simulink model "identifica_srv02l_problem"  (Simulink 7.2)
settings: Solver=ode1  StartTime=0.0  StopTime=3  FixedStep=0.001  RelTol=1e-3  AbsTol=1e-6
values from neighbouring files (symbols this model uses):
  a = param_otim(2)    [calc_all.m]    (also in calc_all_old_v.m; controlador_cal.m = 14.1465; exp1_3.mat = 1; exp1_3_1.mat = 10)
  b = param_otim(1)    [calc_all.m]    (also in calc_all_old_v.m; controlador_cal.m = 4.028; exp1_3.mat = 1; exp1_3_1.mat = 0.825375)
  K_AMP = 1    [exp1_3.mat]    (also in exp1_3_1.mat; exp1_T.mat; exp1_T2.mat; exp1_T3.mat)
  K_ENC = 0.00153398078789    [exp1_3.mat]    (also in exp1_3_1.mat; exp1_T.mat; exp1_T2.mat; exp1_T3.mat)
  K_POT = -0.614355896702    [exp1_3.mat]    (also in exp1_3_1.mat; exp1_T.mat; exp1_T2.mat; exp1_T3.mat)
  K_TACH = -0.99733100114    [exp1_3.mat]    (also in exp1_3_1.mat; exp1_T.mat; exp1_T2.mat; exp1_T3.mat)
  L = 0    [exp1_3.mat]    (also in exp1_3_1.mat = 0.026; exp1_T.mat; exp1_T2.mat; exp1_T3.mat)
  VMAX_AMP = 24    [exp1_3.mat]    (also in exp1_3_1.mat; exp1_T.mat; exp1_T2.mat; exp1_T3.mat)
  VMAX_DAC = 10    [exp1_3.mat]    (also in exp1_3_1.mat; exp1_T.mat; exp1_T2.mat; exp1_T3.mat)
  wcf_e = 157.079632679    [exp1_3.mat]    (also in exp1_3_1.mat; exp1_T.mat; exp1_T2.mat; exp1_T3.mat)
  zetaf_e = 0.9    [exp1_3.mat]    (also in exp1_3_1.mat; exp1_T.mat; exp1_T2.mat; exp1_T3.mat)
undefined symbols (not defined in the file or in its folder): HIL, qc_get_step_size
libraries: quarc_library x4, simulink x1
settings Model: Creator=MLevis  LastModifiedBy=aluno  SimulationMode=external  ExtModeTrigDuration=1000000  BufferReuse=off
settings SolverCC: PositivePriorityOrder=on
settings DataIOCC: LimitDataPoints=off
settings OptimizationCC: BlockReduction=off  BooleanDataType=off  InlineInvariantSignals=on  OptimizeBlockIOStorage=off  BufferReuse=off  ExpressionFolding=off  LocalBlockOutputs=off  InitFltsAndDblsToZero=on
settings DebuggingCC: SaveWithParameterizedLinksMsg=none  SignalResolutionControl=TryResolveAllWithWarning  SolverPrmCheckMsg=none  MultiTaskDSMMsg=warning  MultiTaskCondExecSysMsg=none  StrictBusMsg=None
settings HardwareCC: TargetHWDeviceType=32-bit Generic
settings RTWCC: SystemTargetFile=quarc_windows.tlc  TemplateMakefile=quarc_default_tmf  Description=Quarc Win32 Target  ProcessScript=quarc_windows_make_rtw_hook  IncludeERTFirstTime=on
settings STFCustomTargetCC: TargetFcnLib=ansi_tfl_tmw.mat  TargetPreCompLibLocation=C:\DOCUME~1\ALLUSE~1\DADOSD~1\QUARC\lib\2008b\windows\release  SystemTargetFile=quarc_windows.tlc
settings GRTTargetCC: TargetFcnLib=ansi_tfl_tmw.mat  TargetPreCompLibLocation=C:\DOCUME~1\ALLUSE~1\DADOSD~1\QUARC\lib\2008b\windows\release  CompOptLevelCompliant=off  MatFileLogging=off  ExtMode=on  ExtModeMexFile=quarc_comm

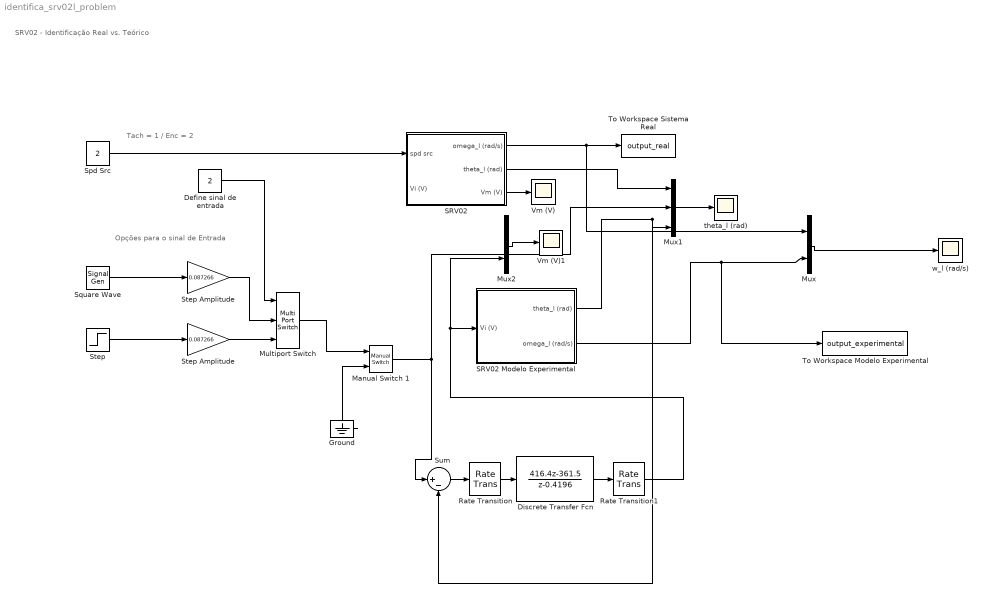
== system identifica_srv02l_problem ==
  note: SRV02 - Identificação
      | Real vs. Teórico
  note: Tach = 1 / Enc = 2
  note: Opções para o sinal de Entrada
  Define sinal de entrada : Constant  Value=2  OutDataType=fixdt(1, 16)  OutScaling=2^0
  Discrete Transfer Fcn : DiscreteTransferFcn  Numerator=[416.4 -361.5]  Denominator=[1 -0.4196]  SampleTime=0.01
  Ground : Ground
  Manual Switch 1 : simulink/Signal Routing/Manual Switch  SystemSampleTime=-1  sw=1  action=0  varsize=off
  Multiport Switch : MultiPortSwitch  Inputs=2  OutDataType=fixdt(1, 16)  OutScaling=2^0
  Mux : Mux  Inputs=2
  Mux1 : Mux  Inputs=3
  Mux2 : Mux  Inputs=2
  Rate Transition : RateTransition  OutPortSampleTime=0.01
  Rate Transition1 : RateTransition  OutPortSampleTime=0.001
  SRV02 : Subsystem
  SRV02 Modelo Experimental : Subsystem
  Spd Src : Constant  Value=2  OutDataType=sfix(16)  OutScaling=2^0
  Square Wave : SignalGenerator  WaveForm=square  Frequency=5
  Step : Step  Time=0.5  SampleTime=0
  Step Amplitude : Gain  Gain=0.087266  ParameterDataType=sfix(16)  ParameterScaling=2^0  OutDataType=sfix(16)  OutScaling=2^0  SaturateOnIntegerOverflow=on  OutDataTypeStr=Inherit: Same as input  ParamDataTypeStr=Inherit: Same as input
  "Step Amplitude " : Gain  Gain=0.087266  ParameterDataType=sfix(16)  ParameterScaling=2^0  OutDataType=sfix(16)  OutScaling=2^0  SaturateOnIntegerOverflow=on  OutDataTypeStr=Inherit: Same as input  ParamDataTypeStr=Inherit: Same as input
  Sum : Sum  Inputs=|+-  OutDataType=sfix(16)  OutScaling=2^0
  To Workspace Modelo Experimental : ToWorkspace  VariableName=output_experimental  SampleTime=-1  SaveFormat=Structure With Time
  To Workspace Sistema Real : ToWorkspace  VariableName=output_real  SampleTime=-1  SaveFormat=Structure With Time
  Vm (V) : Scope
      settings: TimeRange=5  SaveName=Vm  DataFormat=Array
  Vm (V)1 : Scope
      settings: TimeRange=5  SaveName=Vm1  DataFormat=Array
  theta_l (rad) : Scope
      settings: TimeRange=5  YMin=-2.75  YMax=2.75  SaveName=theta  DataFormat=Array
  w_l (rad/s) : Scope
      settings: TimeRange=5  YMin=-2.75  YMax=2.75  SaveName=wl  DataFormat=Array
  wires:
  Mux/1 -> w_l (rad/s)/1
  SRV02/1(omega_l (rad/s)) -> Mux/1, To Workspace Sistema Real/1
  Spd Src/1 -> SRV02/1(spd src)
  Define sinal de entrada/1 -> Multiport Switch/1
  Step/1 -> "Step Amplitude "/1
  Square Wave/1 -> Step Amplitude/1
  "Step Amplitude "/1 -> Multiport Switch/3
  Ground/1 -> Manual Switch 1/2
  SRV02 Modelo Experimental/2(omega_l (rad/s)) -> Mux/2, To Workspace Modelo Experimental/1
  Mux1/1 -> theta_l (rad)/1
  SRV02/2(theta_l (rad)) -> Mux1/1
  SRV02 Modelo Experimental/1(theta_l (rad)) -> Sum/2, Mux1/3
  Multiport Switch/1 -> Manual Switch 1/1
  SRV02/3(Vm (V)) -> Vm (V)/1
  Manual Switch 1/1 -> Sum/1, Mux1/2
  Step Amplitude/1 -> Multiport Switch/2
  Mux2/1 -> Vm (V)1/1
  Sum/1 -> Rate Transition/1
  Rate Transition/1 -> Discrete Transfer Fcn/1
  Discrete Transfer Fcn/1 -> Rate Transition1/1
  Rate Transition1/1 -> SRV02 Modelo Experimental/1(Vi (V)), Mux2/2

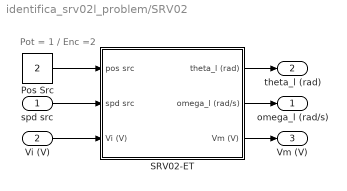
== system identifica_srv02l_problem/SRV02 ==
  note: Pot = 1 / Enc =2
  spd src : Inport  OutDataType=sfix(16)  OutScaling=2^0
  Vi (V) : Inport  Port=2  OutDataType=sfix(16)  OutScaling=2^0
  Pos Src : Constant  Value=2  OutDataType=sfix(16)  OutScaling=2^0
  SRV02-ET : Subsystem
  omega_l (rad/s) : Outport  OutDataType=sfix(16)  OutScaling=2^0
  theta_l (rad) : Outport  Port=2  OutDataType=sfix(16)  OutScaling=2^0
  Vm (V) : Outport  Port=3  OutDataType=sfix(16)  OutScaling=2^0
  wires:
  SRV02-ET/3(Vm (V)) -> Vm (V)/1
  Vi (V)/1 -> SRV02-ET/3(Vi (V))
  SRV02-ET/2(omega_l (rad/s)) -> omega_l (rad/s)/1
  spd src/1 -> SRV02-ET/2(spd src)
  Pos Src/1 -> SRV02-ET/1(pos src)
  SRV02-ET/1(theta_l (rad)) -> theta_l (rad)/1

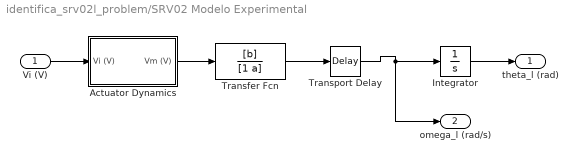
== system identifica_srv02l_problem/SRV02 Modelo Experimental ==
  Vi (V) : Inport  OutDataType=sfix(16)  OutScaling=2^0
  Actuator Dynamics : Subsystem
  Integrator : Integrator
  Transfer Fcn : TransferFcn  Numerator=[b]  Denominator=[1 a]
  Transport Delay : TransportDelay  DelayTime=L
  theta_l (rad) : Outport  OutDataType=sfix(16)  OutScaling=2^0
  omega_l (rad/s) : Outport  Port=2  OutDataType=sfix(16)  OutScaling=2^0
  wires:
  Vi (V)/1 -> Actuator Dynamics/1(Vi (V))
  Actuator Dynamics/1(Vm (V)) -> Transfer Fcn/1
  Integrator/1 -> theta_l (rad)/1
  Transfer Fcn/1 -> Transport Delay/1
  Transport Delay/1 -> Integrator/1, omega_l (rad/s)/1

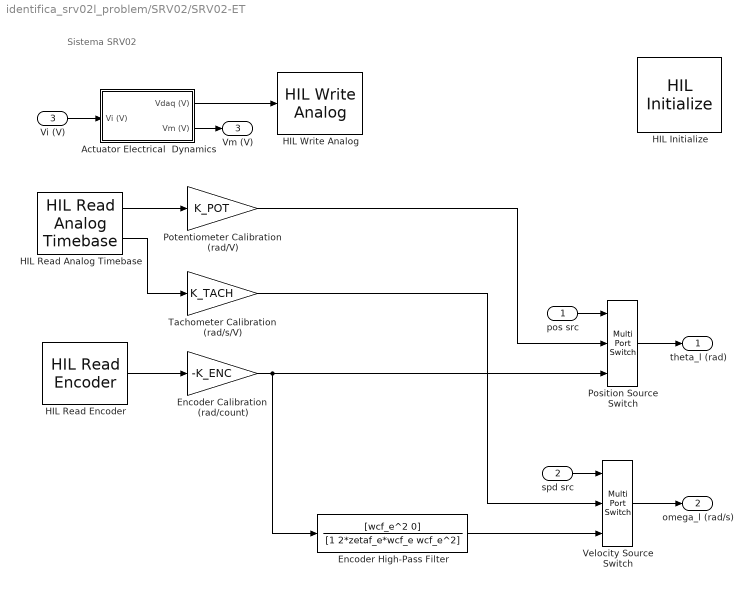
== system identifica_srv02l_problem/SRV02/SRV02-ET ==
  note: Sistema SRV02
  pos src : Inport  OutDataType=sfix(16)  OutScaling=2^0
  spd src : Inport  Port=2  OutDataType=sfix(16)  OutScaling=2^0
  Vi (V) : Inport  Port=3  OutDataType=sfix(16)  OutScaling=2^0
  Actuator Electrical  Dynamics : Subsystem
  Encoder Calibration  (rad/count) : Gain  Gain=-K_ENC  ParameterDataType=sfix(16)  ParameterScaling=2^0  OutDataType=sfix(16)  OutScaling=2^0  SaturateOnIntegerOverflow=on  OutDataTypeStr=Inherit: Same as input  ParamDataTypeStr=Inherit: Same as input
  Encoder High-Pass Filter : TransferFcn  Numerator=[wcf_e^2 0]  Denominator=[1 2*zetaf_e*wcf_e wcf_e^2]
  HIL Initialize : quarc_library/Data Acquisition/Generic/Configuration/HIL Initialize  object_name=HIL-1  board_type=q8_usb  board_number=0  board_options=update_rate=normal  exclusive=off  active=off  hardware_clocks=[0:2]  clock_modes=[]  set_clock_params_at_start=off  set_clock_params_at_switch_in=off  analog_input_channels=[0:7]  analog_input_maximums=10  analog_input_minimums=-10  set_analog_input_params_at_start=on  set_analog_input_params_at_switch_in=off  analog_output_channels=[0:7]  analog_output_maximums=10  analog_output_minimums=-10  initial_analog_outputs=[0]  final_analog_outputs=[0]  watchdog_analog_outputs=0  set_analog_output_params_at_start=on  set_analog_output_params_at_switch_in=off  set_analog_outputs_at_start=on  set_analog_outputs_at_switch_in=off  set_analog_outputs_at_terminate=on  set_analog_outputs_at_switch_out=off  set_analog_outputs_on_watchdog=off  digital_input_channels=[]  digital_output_channels=[0:7]  digital_output_configuration=[]  initial_digital_outputs=[0]  final_digital_outputs=[0]  watchdog_digital_outputs=[0]  set_digital_output_params_at_start=off  set_digital_output_params_at_switch_in=off  set_digital_outputs_at_start=on  set_digital_outputs_at_switch_in=off  set_digital_outputs_at_terminate=on  set_digital_outputs_at_switch_out=off  set_digital_outputs_on_watchdog=off  encoder_channels=[0:7]  quadrature=[4]  encoder_filter_frequency=[]  initial_encoder_counts=[0]  set_encoder_params_at_start=on  set_encoder_params_at_switch_in=off  set_encoder_counts_at_start=on  set_encoder_counts_at_switch_in=off  pwm_channels=[0:7]  pwm_modes=0  pwm_frequency=99.532799999999995e6/4095  pwm_configuration=[0]  pwm_alignment=[0]  pwm_polarity=[1]  pwm_leading_deadband=[0]  pwm_trailing_deadband=[0]  initial_pwm_outputs=[0]  final_pwm_outputs=[0]  watchdog_pwm_outputs=[0]  set_pwm_params_at_start=on  set_pwm_params_at_switch_in=off  set_pwm_outputs_at_start=on  set_pwm_outputs_at_switch_in=off  set_pwm_outputs_at_terminate=on  set_pwm_outputs_at_switch_out=off  set_pwm_outputs_on_watchdog=off  other_output_channels=[]  initial_other_outputs=[]  final_other_outputs=[]  watchdog_other_outputs=[]  set_other_outputs_at_start=off  set_other_outputs_at_switch_in=off  set_other_outputs_at_terminate=off  set_other_outputs_at_switch_out=off  set_other_outputs_on_watchdog=off
  HIL Read Analog Timebase : quarc_library/Data Acquisition/Generic/Timebases/HIL Read Analog Timebase  Tag=unassigned  object_name=HIL-1  clock=0  channels=[0:1]  samples_in_buffer=max(ceil(1/qc_get_step_size), 1)  active=on  vector_output=off
      settings: AttributesFormatString=(%<object_name>)
  HIL Read Encoder : quarc_library/Data Acquisition/Generic/Immediate I//O/HIL Read Encoder  Tag=unassigned  object_name=HIL-1  channels=0  sample_time=qc_get_step_size  active=on  vector_output=off  data_type_mode=Inherit via back propagation  data_type=double
  HIL Write Analog : quarc_library/Data Acquisition/Generic/Immediate I//O/HIL Write Analog  Tag=unassigned  object_name=HIL-1  channels=0  sample_time=-1  active=off  vector_input=off
  Position Source Switch : MultiPortSwitch  Inputs=2
  Potentiometer Calibration  (rad/V) : Gain  Gain=K_POT  ParameterDataType=sfix(16)  ParameterScaling=2^0  OutDataType=sfix(16)  OutScaling=2^0  SaturateOnIntegerOverflow=on  OutDataTypeStr=Inherit: Same as input  ParamDataTypeStr=Inherit: Same as input
  Tachometer Calibration  (rad/s/V) : Gain  Gain=K_TACH  ParameterDataType=sfix(16)  ParameterScaling=2^0  OutDataType=sfix(16)  OutScaling=2^0  SaturateOnIntegerOverflow=on  OutDataTypeStr=Inherit: Same as input  ParamDataTypeStr=Inherit: Same as input
  Velocity Source Switch : MultiPortSwitch  Inputs=2
  theta_l (rad) : Outport  OutDataType=sfix(16)  OutScaling=2^0  InitialOutput=0
  omega_l (rad/s) : Outport  Port=2  OutDataType=sfix(16)  OutScaling=2^0  InitialOutput=0
  Vm (V) : Outport  Port=3  OutDataType=sfix(16)  OutScaling=2^0  InitialOutput=0
  wires:
  HIL Read Analog Timebase/2 -> Tachometer Calibration  (rad/s/V)/1
  HIL Read Encoder/1 -> Encoder Calibration  (rad/count)/1
  Encoder High-Pass Filter/1 -> Velocity Source Switch/3
  Potentiometer Calibration  (rad/V)/1 -> Position Source Switch/2
  spd src/1 -> Velocity Source Switch/1
  pos src/1 -> Position Source Switch/1
  Position Source Switch/1 -> theta_l (rad)/1
  Velocity Source Switch/1 -> omega_l (rad/s)/1
  Actuator Electrical  Dynamics/2(Vm (V)) -> Vm (V)/1
  Actuator Electrical  Dynamics/1(Vdaq (V)) -> HIL Write Analog/1
  HIL Read Analog Timebase/1 -> Potentiometer Calibration  (rad/V)/1
  Vi (V)/1 -> Actuator Electrical  Dynamics/1(Vi (V))
  Encoder Calibration  (rad/count)/1 -> Encoder High-Pass Filter/1, Position Source Switch/3
  Tachometer Calibration  (rad/s/V)/1 -> Velocity Source Switch/2

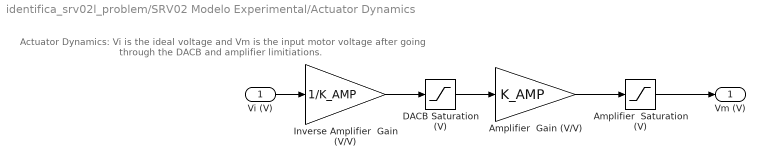
== system identifica_srv02l_problem/SRV02 Modelo Experimental/Actuator Dynamics ==
  note: Actuator Dynamics: Vi is the ideal voltage and Vm is the
      | input motor voltage after going through the DACB and amplifier limitiations.
  Vi (V) : Inport  OutDataType=sfix(16)  OutScaling=2^0
  Amplifier  Gain (V/V) : Gain  Gain=K_AMP  ParameterDataType=sfix(16)  ParameterScaling=2^0  OutDataType=sfix(16)  OutScaling=2^0
  Amplifier  Saturation (V) : Saturate  UpperLimit=VMAX_AMP  LowerLimit=-VMAX_AMP
  DACB Saturation (V) : Saturate  UpperLimit=VMAX_DAC  LowerLimit=-VMAX_DAC
  Inverse Amplifier  Gain (V/V) : Gain  Gain=1/K_AMP  ParameterDataType=sfix(16)  ParameterScaling=2^0  OutDataType=sfix(16)  OutScaling=2^0
  Vm (V) : Outport  OutDataType=sfix(16)  OutScaling=2^0
  wires:
  Inverse Amplifier  Gain (V/V)/1 -> DACB Saturation (V)/1
  DACB Saturation (V)/1 -> Amplifier  Gain (V/V)/1
  Amplifier  Gain (V/V)/1 -> Amplifier  Saturation (V)/1
  Vi (V)/1 -> Inverse Amplifier  Gain (V/V)/1
  Amplifier  Saturation (V)/1 -> Vm (V)/1

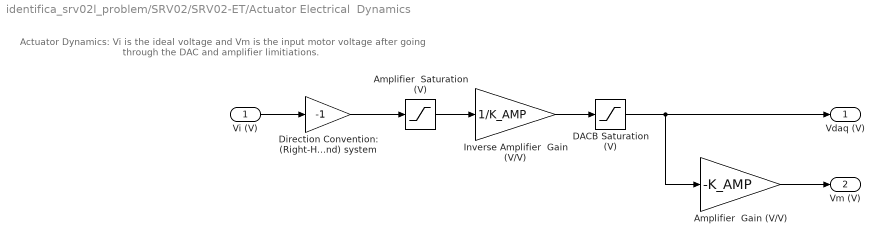
== system identifica_srv02l_problem/SRV02/SRV02-ET/Actuator Electrical  Dynamics ==
  note: Actuator Dynamics: Vi is the ideal voltage and Vm is the
      | input motor voltage after going through the DAC and amplifier limitiations.
  Vi (V) : Inport  OutDataType=sfix(16)  OutScaling=2^0
  Amplifier  Gain (V/V) : Gain  Gain=-K_AMP  ParameterDataType=sfix(16)  ParameterScaling=2^0  OutDataType=sfix(16)  OutScaling=2^0
  Amplifier  Saturation (V) : Saturate  UpperLimit=VMAX_AMP  LowerLimit=-VMAX_AMP
  DACB Saturation (V) : Saturate  UpperLimit=VMAX_DAC  LowerLimit=-VMAX_DAC
  Direction Convention: (Right-Hand) system : Gain  Gain=-1  ParameterDataType=sfix(16)  ParameterScaling=2^0  OutDataType=sfix(16)  OutScaling=2^0  SaturateOnIntegerOverflow=on  OutDataTypeStr=Inherit: Same as input  ParamDataTypeStr=Inherit: Same as input
  Inverse Amplifier  Gain (V/V) : Gain  Gain=1/K_AMP  ParameterDataType=sfix(16)  ParameterScaling=2^0  OutDataType=sfix(16)  OutScaling=2^0
  Vdaq (V) : Outport  OutDataType=sfix(16)  OutScaling=2^0
  Vm (V) : Outport  Port=2  OutDataType=sfix(16)  OutScaling=2^0
  wires:
  Vi (V)/1 -> Direction Convention: (Right-Hand) system/1
  Amplifier  Saturation (V)/1 -> Inverse Amplifier  Gain (V/V)/1
  Inverse Amplifier  Gain (V/V)/1 -> DACB Saturation (V)/1
  DACB Saturation (V)/1 -> Amplifier  Gain (V/V)/1, Vdaq (V)/1
  Amplifier  Gain (V/V)/1 -> Vm (V)/1
  Direction Convention: (Right-Hand) system/1 -> Amplifier  Saturation (V)/1
